simulink model "ModernControlSim"  (Simulink 8.1)
settings: Solver=ode4  StartTime=Tstart  StopTime=Tfinal  FixedStep=Ts  RelTol=1e-3
values from neighbouring files (symbols this model uses):
  A = [0  1  0  0 ... (first row only)    [ModernControlSim.m]
  B = [0 ... (first row only)    [ModernControlSim.m]
  C = [0 0 1 0]    [ModernControlSim.m]
  K = [26.45 0.8325 131.0 31.78]    [ModernControlSim.m]
  L = L'    [ModernControlSim.m]
  N_bar = (b1*K(3)-a2)/b1    [ModernControlSim.m]
undefined symbols (not defined in the file or in its folder): PSD, SIM_XC, Ts, X_START_TIME
libraries: simulink x1
settings Model: Creator=ML-07  LastModifiedBy=econ  BufferReuse=off
settings OptimizationCC: InlineParams=on  BufferReuse=off
settings DebuggingCC: FcnCallInpInsideContextMsg=EnableAllAsWarning  InitInArrayFormatMsg=none
settings GRTTargetCC: CodeReplacementLibrary=None  CPPClassGenCompliant=on

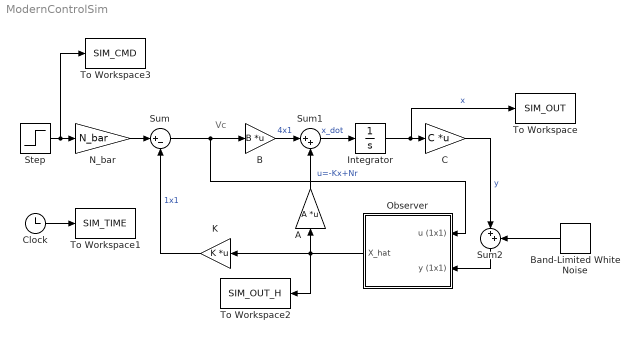
== system ModernControlSim ==
  note: Vc
  A : Gain  Gain=A  Multiplication=Matrix(K*u)
  B : Gain  Gain=B  Multiplication=Matrix(K*u)
  Band-Limited White Noise : simulink/Sources/Band-Limited White Noise  Cov=[PSD]  Ts=Ts  seed=[23341]
  C : Gain  Gain=C  Multiplication=Matrix(K*u)
  Clock : Clock
  Integrator : Integrator
  K : Gain  Gain=K  Multiplication=Matrix(K*u)
  N_bar : Gain  Gain=N_bar
  Observer : Subsystem
  Step : Step  Time=X_START_TIME  After=SIM_XC  SampleTime=0
  Sum : Sum  Inputs=|+-
  Sum1 : Sum  Inputs=|++
  Sum2 : Sum  Inputs=|++
  To Workspace : ToWorkspace  VariableName=SIM_OUT  SampleTime=-1
  To Workspace1 : ToWorkspace  VariableName=SIM_TIME  SampleTime=-1
  To Workspace2 : ToWorkspace  VariableName=SIM_OUT_H  SampleTime=-1
  To Workspace3 : ToWorkspace  VariableName=SIM_CMD  SampleTime=-1
  wires:
  Sum1/1 -> Integrator/1  "x_dot"
  Integrator/1 -> To Workspace/1, C/1  "x"
  A/1 -> Sum1/2
  B/1 -> Sum1/1  "4x1"
  K/1 -> Sum/2  "1x1"
  Clock/1 -> To Workspace1/1
  Step/1 -> To Workspace3/1, N_bar/1
  N_bar/1 -> Sum/1
  C/1 -> Sum2/1  "y"
  Observer/1(X_hat) -> A/1, K/1, To Workspace2/1
  Sum/1 -> B/1, Observer/1(u (1x1))  "u=-Kx+Nr"
  Sum2/1 -> Observer/2(y (1x1))
  Band-Limited White Noise/1 -> Sum2/2

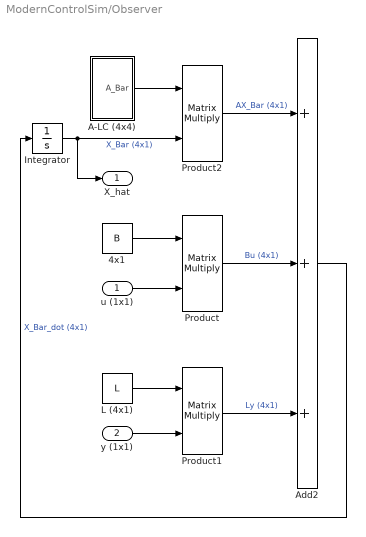
== system ModernControlSim/Observer ==
  u (1x1) : Inport
  y (1x1) : Inport  Port=2
  4x1 : Constant  Value=B  VectorParams1D=off
  A-LC (4x4) : Subsystem
  Add2 : Sum  Inputs=+++
  Integrator : Integrator
  L (4x1) : Constant  Value=L  VectorParams1D=off
  Product : Product  Multiplication=Matrix(*)
  Product1 : Product  Multiplication=Matrix(*)
  Product2 : Product  Multiplication=Matrix(*)
  X_hat : Outport
  wires:
  u (1x1)/1 -> Product/2
  L (4x1)/1 -> Product1/1
  y (1x1)/1 -> Product1/2
  Product2/1 -> Add2/1  "AX_Bar (4x1)"
  Product/1 -> Add2/2  "Bu (4x1)"
  Product1/1 -> Add2/3  "Ly (4x1)"
  Add2/1 -> Integrator/1  "X_Bar_dot (4x1)"
  Integrator/1 -> X_hat/1, Product2/2  "X_Bar (4x1)"
  A-LC (4x4)/1(A_Bar) -> Product2/1
  4x1/1 -> Product/1

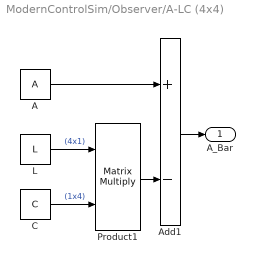
== system ModernControlSim/Observer/A-LC (4x4) ==
  A : Constant  Value=A  VectorParams1D=off
  Add1 : Sum  Inputs=+-
  C : Constant  Value=C  VectorParams1D=off
  L : Constant  Value=L  VectorParams1D=off
  Product1 : Product  Multiplication=Matrix(*)
  A_Bar : Outport
  wires:
  Product1/1 -> Add1/2
  A/1 -> Add1/1
  Add1/1 -> A_Bar/1
  L/1 -> Product1/1  "(4x1)"
  C/1 -> Product1/2  "(1x4)"
